simulink model "LinkageC"  (R2025b)
settings: Solver=VariableStepAuto  StartTime=0  StopTime=numPeriods*T  RelTol=1e-3  AbsTol=1e-3
values from neighbouring files (symbols this model uses):
  A_G = 56.801    [LinkageGeometrySetUp.m]    (also in LinkageGeometrySetUp_imp.m = 55; LinkageGeometry_Fabio_ver.m = 20)
  alpha_0 = deg2rad(0.5)    [Iteration.m]    (also in Iteration_geometry.m; StartUp.m)
  alpha_stall_static = deg2rad(13)    [Iteration.m]    (also in Iteration_geometry.m; StartUp.m)
  AR = b^2/A    [LinkageGeometry_Modify.m]    (also in StartUp.m)
  Cd_cf = 1.5    [Iteration.m]    (also in Iteration_geometry.m; StartUp.m)
  CordOut = linspace(CordOut_root, CordOut_tip, WingSecNum_Out)    [LinkageGeometry_Modify.m]    (also in StartUp.m)
  D = 0;" newline      "    return;" newline      "end" newline      "q = 0.5*rho*Vmag^2;" newline      "D = q*S*CD;" newline      "L = q*S*CL;" newline      "    [build_wing_template.m]
  del_t = t_tot/(numSample)    [InputSetUp.m]
  eta_s = 0.90    (= 0.9)    [Iteration.m]    (also in Iteration_geometry.m; StartUp.m)
  InboardCord = 0.35*L_D/0.037    [LinkageGeometry_Modify.m]    (also in StartUp.m = 0.4)
  k_inboard = k * InboardCord/meanCord    [LinkageGeometry_Modify.m]    (also in StartUp.m = 12.5663706144)
  k_outboard = k * CordOut/meanCord    [LinkageGeometry_Modify.m]    (also in StartUp.m)
  Ka = 10    [StartUp3_control.m]
  Km = 73    [StartUp3_control.m]
  L_C = (3.589/1.5)*L_D    [LinkageGeometrySetUp.m]    (also in LinkageGeometrySetUp_imp.m = (9.37/3.7)*L_D; LinkageGeometry_Fabio_ver.m = 0.07885)
  L_C1 = (2.445/1.5)*L_D    [LinkageGeometrySetUp.m]    (also in LinkageGeometrySetUp_imp.m = (5.91/3.7)*L_D; LinkageGeometry_Fabio_ver.m = 0.04893)
  L_D = L_D_val(iter)    [Iteration_geometry.m]    (also in LinkageGeometry_Fabio_ver.m = 0.03019; StartUp.m = 0.037)
  L_EF = (1.494/1.5)*L_D    [LinkageGeometrySetUp.m]    (also in LinkageGeometrySetUp_imp.m = (4.468/3.7)*L_D; LinkageGeometry_Fabio_ver.m = 0.036)
  L_EG = (1.265/1.5)*L_D    [LinkageGeometrySetUp.m]    (also in LinkageGeometrySetUp_imp.m = L_C2; LinkageGeometry_Fabio_ver.m = 0.03)
  L_F = (16.189/1.5)*L_D    [LinkageGeometrySetUp.m]    (also in LinkageGeometrySetUp_imp.m = (39.93/3.7)*L_D; LinkageGeometry_Fabio_ver.m = 0.364)
  L_FH = (1.002/1.5)*L_D    [LinkageGeometrySetUp.m]    (also in LinkageGeometrySetUp_imp.m = (2.842/3.7)*L_D; LinkageGeometry_Fabio_ver.m = 0.02)
  L_Fl = (16.118/1.5)*L_D    [LinkageGeometrySetUp.m]    (also in LinkageGeometrySetUp_imp.m = L_F; LinkageGeometry_Fabio_ver.m = 0.364)
  L_Fp = (4.051/1.5)*L_D    [LinkageGeometrySetUp.m]    (also in LinkageGeometrySetUp_imp.m = (9.99/3.7)*L_D; LinkageGeometry_Fabio_ver.m = 0.14288)
  L_GH = (1.129/1.5)*L_D    [LinkageGeometrySetUp.m]    (also in LinkageGeometrySetUp_imp.m = (3.046/3.7)*L_D; LinkageGeometry_Fabio_ver.m = 0.016)
  L_t = 0.5/100    (= 0.005)    [LinkageGeometrySetUp.m]    (also in LinkageGeometrySetUp_imp.m; LinkageGeometry_Fabio_ver.m; LinkageGeometry_Modify.m)
  L_tip = (19.334/1.5)*L_D    [LinkageGeometrySetUp.m]    (also in LinkageGeometrySetUp_imp.m = (43/3.7)*L_D; LinkageGeometry_Fabio_ver.m = 0.55)
  M_in_i = M_in/WingSecNum_In    (= 0.0341666666667)    [StartUp.m]
  M_ser = 0.02    [StartUp.m]
  mu = 1.81e-5    (= 1.81e-05)    [Iteration.m]    (also in Iteration_geometry.m; StartUp.m)
  noise_freq_cutoff = 20*ang_freq    [InputSetUp.m]
  P_ref = 10    [StartUp3_control.m]
  phase_data_lookup = phase_data_lookup(1:(end-1))    [StartUp.m]
  pitch_data_lookup = pitch_ts.Data(1:numSampPerT)    [InputSetUp.m]
  pitch_gain = linspace(0.1, 1, WingSecNum_Out)    [InputSetUp.m]
  pitch_lookup_input = 1    [Iteration.m]    (also in Iteration_geometry.m; StartUp.m)
  pitch_mean = deg2rad(20)    [Iteration.m]    (also in Iteration_geometry.m; Iteration_speed.m; StartUp.m = deg2rad(1); StartUp3_control.m = deg2rad(1))
  rho = 1.225    [StartUp.m]
  SectionWidth_In = L_Inboard/WingSecNum_In    [LinkageGeometry_Modify.m]    (also in StartUp.m = (L_Inboard/WingSecNum_In)*0.6)
  SectionWidth_Out = L_outboard/WingSecNum_Out    [LinkageGeometry_Modify.m]    (also in StartUp.m)
  SpeedControlYes = 1    [StartUp3_control.m]
  TorqueLimit = 7.2    [StartUp3_control.m]
  U = 0.1    [Iteration.m]    (also in Iteration_geometry.m; StartUp.m)
  xi = 0.0    (= 0)    [Iteration.m]    (also in Iteration_geometry.m; StartUp.m)
undefined symbols (not defined in the file or in its folder): angle_data_lookup, DiscIntNeverNeededParam, magnitude, Pivot, X, Y, Z
libraries: sm_lib x1370, nesl_utility x916, simulink x478, cstblocks x78, simulink_extras x10, slpidlib x2
(part 53 of 57)

== matlab function LinkageC/Subsystem2/Parallelogram/WingSeg_In_2/1993dL&dT/AeroCalc ==
  data: dL output size=[1 1]; R input size=[3 3]; dT output size=[1 1]; h_dot input size=[1 1]; h_ddot input size=[1 1]; i input size=[1 1]; in input size=[1 1]; pitch_i input size=[1 1]; pitch_i_d input size=[1 1]; pitch_i_dd input size=[1 1]; pitch_mean parameter size=[1 1]; pitch_gain parameter; k_inboard parameter; k_outboard parameter; U parameter size=[1 1]; rho parameter size=[1 1]; AR parameter size=[1 1]; mu parameter size=[1 1]; xi parameter size=[1 1]; alpha_0 parameter size=[1 1]; alpha_stall_static parameter size=[1 1]; eta_s parameter size=[1 1]; Cd_cf parameter size=[1 1]; InboardCord parameter; CordOut parameter; SectionWidth_In parameter; SectionWidth_Out parameter size=[1 1]; stall_yes output
function [dL, dT, stall_yes] = fcn(R, h_dot, h_ddot, i, in , ...
    pitch_i,pitch_i_d,pitch_i_dd, pitch_mean, pitch_gain, ...
    k_inboard, k_outboard, ...
    U,rho, AR, mu, xi, alpha_0, alpha_stall_static, eta_s, Cd_cf, ...
    InboardCord,CordOut, SectionWidth_In,SectionWidth_Out) 
    % Notes:
    %   - wing root i = 1, wing tip i = wing section number
    %   - the smaller the i, the closer to the root
    % Parameters:
    %   - R = rotational matrix
    %   - h_dot = leading edge velocity (m/s)
    %   - pitch (may be inaccurate, but currently taken as w.r.t spar....)

    R = 1*R;  % rotation matrix (not yet used)
     
    % Simple steady state version (?):
    % V = [Vx, Vy, Vz];
    % Vmag = norm(V);
    % if Vmag < 1e-9
    %     Fx = 0; Fy = 0; Fz = 0; L = 0; D = 0;
    %     return;
    % end
    % q = 0.5*rho*Vmag^2;
    % D = q*S*CD;
    % L = q*S*CL;
    % % drag opposite velocity, lift along +y 
    % % U is in + z direction
    % u = (V+[0,0,U]) / Vmag; % normal vector for V direction relative to air
    % Fdrag = -D*u;
    % Flift = [0,L,0];
    % F = Fdrag + Flift;
    % Fx = F(1); Fy = F(2); Fz = F(3);


    % 1993 code start's here --------------------------------------------
    i = round(i);
    C_1 = 0.5*AR/(2.32+AR);
    C_2 = 0.181+0.772/AR;
    F_k = @(k)   1 - C_1 *(k.^2)./(k.^2 +C_2^2);
    G_k = @(k)   -C_1*C_2*k./(k.^2 +C_2^2);
    C_k = @(k)   F_k(k) + 1i*G_k(k);

    if (round(in) == 1)
        % when it's inboard wing
        dy = SectionWidth_In;
        cord_i = InboardCord;
        pitch_gain_i = 0;
        k_i = k_inboard;
        %C_k_Jones_i = C_k_Jones(k_inboard);
    else % in == 0
        % when it's outboard wing
        dy = SectionWidth_Out;
        cord_i = CordOut(i);
        pitch_gain_i = pitch_gain(i);
        k_i = k_outboard(i);
        %C_k_Jones_i = C_k_Jones(k_outboard(i));
    end

    % scaling the pitch angle
    pitch_mean_i = pitch_mean; % pitch mean is same for all. though not 
                               % shown in simulation for inboard arm
    pitch_i    = pitch_i   *pitch_gain_i;
    pitch_i_d  = pitch_i_d *pitch_gain_i;
    pitch_i_dd = pitch_i_dd*pitch_gain_i;

    w0_U = 2*(alpha_0 + pitch_mean_i)/ (2+AR);

    %all pitch values are in rad
    alpha_i = (h_dot * cos(pitch_i) ...
               + 0.75 * cord_i * pitch_i_d ...
               + U * (pitch_i - pitch_mean_i))/U;
        
    % Time derivative of alpha_i
    alpha_i_d = (h_ddot * cos(pitch_i) ...
            - h_dot * sin(pitch_i) * pitch_i_d ...
            + 0.75 * cord_i * pitch_i_dd ...
            + U * pitch_i_d ) / U;

    %alpha_prime = C_k_Jones_i*alpha_i - w0_U;
    % assume sinusoidal pitching, then:
    alpha_prime = (AR/(2+AR))*(F_k(k_i)*alpha_i + cord_i*G_k(k_i)*alpha_i_d/(2*U*k_i))- w0_U;
    %alpha_prime = alpha_i - w0_U;

    V_34_term1 = U*cos(pitch_i) - h_dot*sin(pitch_i);
    V_34_term2 = U*(alpha_prime+pitch_mean_i) - 0.5*cord_i*pitch_i_d;
    V_34 = sqrt(V_34_term1^2 + V_34_term2^2);

    Cn_y = 2 * pi * (alpha_prime + alpha_0 + pitch_mean_i);
   
    dNc = 0.5*rho*U*V_34*Cn_y*cord_i*dy;

    V_24_d =  U * alpha_i_d - 0.25 * cord_i * pitch_i_dd;
    dNa = 0.25*rho*pi*(cord_i^2)*V_24_d*dy;

    dN = dNa + dNc;

    % Eq. (17): chordwise force due to camber
    dD_camber = -2*pi*alpha_0*(alpha_prime + pitch_mean_i) ...
                * (rho*U*V_34/2) * cord_i * dy;

    % Eq. (18): leading-edge suction term
    dT_s = eta_s * 2*pi * ( alpha_prime + pitch_mean_i ...
          - (cord_i*pitch_i_d)/(4*U) )^2 ...
          * (rho*U*V_34/2) * cord_i * dy;
    
    % Eq. (19): viscous skin-friction drag
    % Eq. (20): tangential flow speed approximation
    V_x = U*cos(pitch_i) - h_dot*sin(pitch_i);
    
    Re_i   = rho * V_34 * cord_i / mu;
    c_df_i = 0.89 / (log10(Re_i)^2.58);
    dD_f = c_df_i * (rho*V_x^2/2) * cord_i * dy;
    
    % Eq. (21): total chordwise force
    dFx = dT_s - dD_camber - dD_f;
    
    % Eq. (22): dynamic stall angle
    alpha_stall = alpha_stall_static + xi * sqrt(abs(cord_i * pitch_i_d / (2*U)));

    % Eq. (23)
    stall_metric = alpha_prime + pitch_mean_i - 0.75 * (cord_i * pitch_i_d / U);
    stall_yes = stall_metric - alpha_stall; 
    if stall_yes > 0
        V_n = h_dot*cos(pitch_i) + 0.5*cord_i*pitch_i_d + U*sin(pitch_i);
        V_hat = sqrt(V_x^2 + V_n^2);
  
        dNc_sep = Cd_cf * 0.5 * rho * V_hat * V_n * cord_i * dy;
        dNa_sep = 0.5*dNa;

        dN = dNc_sep + dNa_sep;
        dFx = 0;  
    end
    
    dL = dN * cos(pitch_i) + dFx * sin(pitch_i);
    dT = dFx * cos(pitch_i) - dN * sin(pitch_i);
end

== matlab function LinkageC/Subsystem2/Parallelogram/WingSeg_In_3/1993dL&dT/AeroCalc ==
  data: dL output size=[1 1]; R input size=[3 3]; dT output size=[1 1]; h_dot input size=[1 1]; h_ddot input size=[1 1]; i input size=[1 1]; in input size=[1 1]; pitch_i input size=[1 1]; pitch_i_d input size=[1 1]; pitch_i_dd input size=[1 1]; pitch_mean parameter size=[1 1]; pitch_gain parameter; k_inboard parameter; k_outboard parameter; U parameter size=[1 1]; rho parameter size=[1 1]; AR parameter size=[1 1]; mu parameter size=[1 1]; xi parameter size=[1 1]; alpha_0 parameter size=[1 1]; alpha_stall_static parameter size=[1 1]; eta_s parameter size=[1 1]; Cd_cf parameter size=[1 1]; InboardCord parameter; CordOut parameter; SectionWidth_In parameter; SectionWidth_Out parameter size=[1 1]; stall_yes output
function [dL, dT, stall_yes] = fcn(R, h_dot, h_ddot, i, in , ...
    pitch_i,pitch_i_d,pitch_i_dd, pitch_mean, pitch_gain, ...
    k_inboard, k_outboard, ...
    U,rho, AR, mu, xi, alpha_0, alpha_stall_static, eta_s, Cd_cf, ...
    InboardCord,CordOut, SectionWidth_In,SectionWidth_Out) 
    % Notes:
    %   - wing root i = 1, wing tip i = wing section number
    %   - the smaller the i, the closer to the root
    % Parameters:
    %   - R = rotational matrix
    %   - h_dot = leading edge velocity (m/s)
    %   - pitch (may be inaccurate, but currently taken as w.r.t spar....)

    R = 1*R;  % rotation matrix (not yet used)
     
    % Simple steady state version (?):
    % V = [Vx, Vy, Vz];
    % Vmag = norm(V);
    % if Vmag < 1e-9
    %     Fx = 0; Fy = 0; Fz = 0; L = 0; D = 0;
    %     return;
    % end
    % q = 0.5*rho*Vmag^2;
    % D = q*S*CD;
    % L = q*S*CL;
    % % drag opposite velocity, lift along +y 
    % % U is in + z direction
    % u = (V+[0,0,U]) / Vmag; % normal vector for V direction relative to air
    % Fdrag = -D*u;
    % Flift = [0,L,0];
    % F = Fdrag + Flift;
    % Fx = F(1); Fy = F(2); Fz = F(3);


    % 1993 code start's here --------------------------------------------
    i = round(i);
    C_1 = 0.5*AR/(2.32+AR);
    C_2 = 0.181+0.772/AR;
    F_k = @(k)   1 - C_1 *(k.^2)./(k.^2 +C_2^2);
    G_k = @(k)   -C_1*C_2*k./(k.^2 +C_2^2);
    C_k = @(k)   F_k(k) + 1i*G_k(k);

    if (round(in) == 1)
        % when it's inboard wing
        dy = SectionWidth_In;
        cord_i = InboardCord;
        pitch_gain_i = 0;
        k_i = k_inboard;
        %C_k_Jones_i = C_k_Jones(k_inboard);
    else % in == 0
        % when it's outboard wing
        dy = SectionWidth_Out;
        cord_i = CordOut(i);
        pitch_gain_i = pitch_gain(i);
        k_i = k_outboard(i);
        %C_k_Jones_i = C_k_Jones(k_outboard(i));
    end

    % scaling the pitch angle
    pitch_mean_i = pitch_mean; % pitch mean is same for all. though not 
                               % shown in simulation for inboard arm
    pitch_i    = pitch_i   *pitch_gain_i;
    pitch_i_d  = pitch_i_d *pitch_gain_i;
    pitch_i_dd = pitch_i_dd*pitch_gain_i;

    w0_U = 2*(alpha_0 + pitch_mean_i)/ (2+AR);

    %all pitch values are in rad
    alpha_i = (h_dot * cos(pitch_i) ...
               + 0.75 * cord_i * pitch_i_d ...
               + U * (pitch_i - pitch_mean_i))/U;
        
    % Time derivative of alpha_i
    alpha_i_d = (h_ddot * cos(pitch_i) ...
            - h_dot * sin(pitch_i) * pitch_i_d ...
            + 0.75 * cord_i * pitch_i_dd ...
            + U * pitch_i_d ) / U;

    %alpha_prime = C_k_Jones_i*alpha_i - w0_U;
    % assume sinusoidal pitching, then:
    alpha_prime = (AR/(2+AR))*(F_k(k_i)*alpha_i + cord_i*G_k(k_i)*alpha_i_d/(2*U*k_i))- w0_U;
    %alpha_prime = alpha_i - w0_U;

    V_34_term1 = U*cos(pitch_i) - h_dot*sin(pitch_i);
    V_34_term2 = U*(alpha_prime+pitch_mean_i) - 0.5*cord_i*pitch_i_d;
    V_34 = sqrt(V_34_term1^2 + V_34_term2^2);

    Cn_y = 2 * pi * (alpha_prime + alpha_0 + pitch_mean_i);
   
    dNc = 0.5*rho*U*V_34*Cn_y*cord_i*dy;

    V_24_d =  U * alpha_i_d - 0.25 * cord_i * pitch_i_dd;
    dNa = 0.25*rho*pi*(cord_i^2)*V_24_d*dy;

    dN = dNa + dNc;

    % Eq. (17): chordwise force due to camber
    dD_camber = -2*pi*alpha_0*(alpha_prime + pitch_mean_i) ...
                * (rho*U*V_34/2) * cord_i * dy;

    % Eq. (18): leading-edge suction term
    dT_s = eta_s * 2*pi * ( alpha_prime + pitch_mean_i ...
          - (cord_i*pitch_i_d)/(4*U) )^2 ...
          * (rho*U*V_34/2) * cord_i * dy;
    
    % Eq. (19): viscous skin-friction drag
    % Eq. (20): tangential flow speed approximation
    V_x = U*cos(pitch_i) - h_dot*sin(pitch_i);
    
    Re_i   = rho * V_34 * cord_i / mu;
    c_df_i = 0.89 / (log10(Re_i)^2.58);
    dD_f = c_df_i * (rho*V_x^2/2) * cord_i * dy;
    
    % Eq. (21): total chordwise force
    dFx = dT_s - dD_camber - dD_f;
    
    % Eq. (22): dynamic stall angle
    alpha_stall = alpha_stall_static + xi * sqrt(abs(cord_i * pitch_i_d / (2*U)));

    % Eq. (23)
    stall_metric = alpha_prime + pitch_mean_i - 0.75 * (cord_i * pitch_i_d / U);
    stall_yes = stall_metric - alpha_stall; 
    if stall_yes > 0
        V_n = h_dot*cos(pitch_i) + 0.5*cord_i*pitch_i_d + U*sin(pitch_i);
        V_hat = sqrt(V_x^2 + V_n^2);
  
        dNc_sep = Cd_cf * 0.5 * rho * V_hat * V_n * cord_i * dy;
        dNa_sep = 0.5*dNa;

        dN = dNc_sep + dNa_sep;
        dFx = 0;  
    end
    
    dL = dN * cos(pitch_i) + dFx * sin(pitch_i);
    dT = dFx * cos(pitch_i) - dN * sin(pitch_i);
end

== matlab function LinkageC/Subsystem2/Parallelogram/WingSeg_In_4/1993dL&dT/AeroCalc ==
  data: dL output size=[1 1]; R input size=[3 3]; dT output size=[1 1]; h_dot input size=[1 1]; h_ddot input size=[1 1]; i input size=[1 1]; in input size=[1 1]; pitch_i input size=[1 1]; pitch_i_d input size=[1 1]; pitch_i_dd input size=[1 1]; pitch_mean parameter size=[1 1]; pitch_gain parameter; k_inboard parameter; k_outboard parameter; U parameter size=[1 1]; rho parameter size=[1 1]; AR parameter size=[1 1]; mu parameter size=[1 1]; xi parameter size=[1 1]; alpha_0 parameter size=[1 1]; alpha_stall_static parameter size=[1 1]; eta_s parameter size=[1 1]; Cd_cf parameter size=[1 1]; InboardCord parameter; CordOut parameter; SectionWidth_In parameter; SectionWidth_Out parameter size=[1 1]; stall_yes output
function [dL, dT, stall_yes] = fcn(R, h_dot, h_ddot, i, in , ...
    pitch_i,pitch_i_d,pitch_i_dd, pitch_mean, pitch_gain, ...
    k_inboard, k_outboard, ...
    U,rho, AR, mu, xi, alpha_0, alpha_stall_static, eta_s, Cd_cf, ...
    InboardCord,CordOut, SectionWidth_In,SectionWidth_Out) 
    % Notes:
    %   - wing root i = 1, wing tip i = wing section number
    %   - the smaller the i, the closer to the root
    % Parameters:
    %   - R = rotational matrix
    %   - h_dot = leading edge velocity (m/s)
    %   - pitch (may be inaccurate, but currently taken as w.r.t spar....)

    R = 1*R;  % rotation matrix (not yet used)
     
    % Simple steady state version (?):
    % V = [Vx, Vy, Vz];
    % Vmag = norm(V);
    % if Vmag < 1e-9
    %     Fx = 0; Fy = 0; Fz = 0; L = 0; D = 0;
    %     return;
    % end
    % q = 0.5*rho*Vmag^2;
    % D = q*S*CD;
    % L = q*S*CL;
    % % drag opposite velocity, lift along +y 
    % % U is in + z direction
    % u = (V+[0,0,U]) / Vmag; % normal vector for V direction relative to air
    % Fdrag = -D*u;
    % Flift = [0,L,0];
    % F = Fdrag + Flift;
    % Fx = F(1); Fy = F(2); Fz = F(3);


    % 1993 code start's here --------------------------------------------
    i = round(i);
    C_1 = 0.5*AR/(2.32+AR);
    C_2 = 0.181+0.772/AR;
    F_k = @(k)   1 - C_1 *(k.^2)./(k.^2 +C_2^2);
    G_k = @(k)   -C_1*C_2*k./(k.^2 +C_2^2);
    C_k = @(k)   F_k(k) + 1i*G_k(k);

    if (round(in) == 1)
        % when it's inboard wing
        dy = SectionWidth_In;
        cord_i = InboardCord;
        pitch_gain_i = 0;
        k_i = k_inboard;
        %C_k_Jones_i = C_k_Jones(k_inboard);
    else % in == 0
        % when it's outboard wing
        dy = SectionWidth_Out;
        cord_i = CordOut(i);
        pitch_gain_i = pitch_gain(i);
        k_i = k_outboard(i);
        %C_k_Jones_i = C_k_Jones(k_outboard(i));
    end

    % scaling the pitch angle
    pitch_mean_i = pitch_mean; % pitch mean is same for all. though not 
                               % shown in simulation for inboard arm
    pitch_i    = pitch_i   *pitch_gain_i;
    pitch_i_d  = pitch_i_d *pitch_gain_i;
    pitch_i_dd = pitch_i_dd*pitch_gain_i;

    w0_U = 2*(alpha_0 + pitch_mean_i)/ (2+AR);

    %all pitch values are in rad
    alpha_i = (h_dot * cos(pitch_i) ...
               + 0.75 * cord_i * pitch_i_d ...
               + U * (pitch_i - pitch_mean_i))/U;
        
    % Time derivative of alpha_i
    alpha_i_d = (h_ddot * cos(pitch_i) ...
            - h_dot * sin(pitch_i) * pitch_i_d ...
            + 0.75 * cord_i * pitch_i_dd ...
            + U * pitch_i_d ) / U;

    %alpha_prime = C_k_Jones_i*alpha_i - w0_U;
    % assume sinusoidal pitching, then:
    alpha_prime = (AR/(2+AR))*(F_k(k_i)*alpha_i + cord_i*G_k(k_i)*alpha_i_d/(2*U*k_i))- w0_U;
    %alpha_prime = alpha_i - w0_U;

    V_34_term1 = U*cos(pitch_i) - h_dot*sin(pitch_i);
    V_34_term2 = U*(alpha_prime+pitch_mean_i) - 0.5*cord_i*pitch_i_d;
    V_34 = sqrt(V_34_term1^2 + V_34_term2^2);

    Cn_y = 2 * pi * (alpha_prime + alpha_0 + pitch_mean_i);
   
    dNc = 0.5*rho*U*V_34*Cn_y*cord_i*dy;

    V_24_d =  U * alpha_i_d - 0.25 * cord_i * pitch_i_dd;
    dNa = 0.25*rho*pi*(cord_i^2)*V_24_d*dy;

    dN = dNa + dNc;

    % Eq. (17): chordwise force due to camber
    dD_camber = -2*pi*alpha_0*(alpha_prime + pitch_mean_i) ...
                * (rho*U*V_34/2) * cord_i * dy;

    % Eq. (18): leading-edge suction term
    dT_s = eta_s * 2*pi * ( alpha_prime + pitch_mean_i ...
          - (cord_i*pitch_i_d)/(4*U) )^2 ...
          * (rho*U*V_34/2) * cord_i * dy;
    
    % Eq. (19): viscous skin-friction drag
    % Eq. (20): tangential flow speed approximation
    V_x = U*cos(pitch_i) - h_dot*sin(pitch_i);
    
    Re_i   = rho * V_34 * cord_i / mu;
    c_df_i = 0.89 / (log10(Re_i)^2.58);
    dD_f = c_df_i * (rho*V_x^2/2) * cord_i * dy;
    
    % Eq. (21): total chordwise force
    dFx = dT_s - dD_camber - dD_f;
    
    % Eq. (22): dynamic stall angle
    alpha_stall = alpha_stall_static + xi * sqrt(abs(cord_i * pitch_i_d / (2*U)));

    % Eq. (23)
    stall_metric = alpha_prime + pitch_mean_i - 0.75 * (cord_i * pitch_i_d / U);
    stall_yes = stall_metric - alpha_stall; 
    if stall_yes > 0
        V_n = h_dot*cos(pitch_i) + 0.5*cord_i*pitch_i_d + U*sin(pitch_i);
        V_hat = sqrt(V_x^2 + V_n^2);
  
        dNc_sep = Cd_cf * 0.5 * rho * V_hat * V_n * cord_i * dy;
        dNa_sep = 0.5*dNa;

        dN = dNc_sep + dNa_sep;
        dFx = 0;  
    end
    
    dL = dN * cos(pitch_i) + dFx * sin(pitch_i);
    dT = dFx * cos(pitch_i) - dN * sin(pitch_i);
end

== matlab function LinkageC/Subsystem2/Parallelogram/WingSeg_In_5/1993dL&dT/AeroCalc ==
  data: dL output size=[1 1]; R input size=[3 3]; dT output size=[1 1]; h_dot input size=[1 1]; h_ddot input size=[1 1]; i input size=[1 1]; in input size=[1 1]; pitch_i input size=[1 1]; pitch_i_d input size=[1 1]; pitch_i_dd input size=[1 1]; pitch_mean parameter size=[1 1]; pitch_gain parameter; k_inboard parameter; k_outboard parameter; U parameter size=[1 1]; rho parameter size=[1 1]; AR parameter size=[1 1]; mu parameter size=[1 1]; xi parameter size=[1 1]; alpha_0 parameter size=[1 1]; alpha_stall_static parameter size=[1 1]; eta_s parameter size=[1 1]; Cd_cf parameter size=[1 1]; InboardCord parameter; CordOut parameter; SectionWidth_In parameter; SectionWidth_Out parameter size=[1 1]; stall_yes output
function [dL, dT, stall_yes] = fcn(R, h_dot, h_ddot, i, in , ...
    pitch_i,pitch_i_d,pitch_i_dd, pitch_mean, pitch_gain, ...
    k_inboard, k_outboard, ...
    U,rho, AR, mu, xi, alpha_0, alpha_stall_static, eta_s, Cd_cf, ...
    InboardCord,CordOut, SectionWidth_In,SectionWidth_Out) 
    % Notes:
    %   - wing root i = 1, wing tip i = wing section number
    %   - the smaller the i, the closer to the root
    % Parameters:
    %   - R = rotational matrix
    %   - h_dot = leading edge velocity (m/s)
    %   - pitch (may be inaccurate, but currently taken as w.r.t spar....)

    R = 1*R;  % rotation matrix (not yet used)
     
    % Simple steady state version (?):
    % V = [Vx, Vy, Vz];
    % Vmag = norm(V);
    % if Vmag < 1e-9
    %     Fx = 0; Fy = 0; Fz = 0; L = 0; D = 0;
    %     return;
    % end
    % q = 0.5*rho*Vmag^2;
    % D = q*S*CD;
    % L = q*S*CL;
    % % drag opposite velocity, lift along +y 
    % % U is in + z direction
    % u = (V+[0,0,U]) / Vmag; % normal vector for V direction relative to air
    % Fdrag = -D*u;
    % Flift = [0,L,0];
    % F = Fdrag + Flift;
    % Fx = F(1); Fy = F(2); Fz = F(3);


    % 1993 code start's here --------------------------------------------
    i = round(i);
    C_1 = 0.5*AR/(2.32+AR);
    C_2 = 0.181+0.772/AR;
    F_k = @(k)   1 - C_1 *(k.^2)./(k.^2 +C_2^2);
    G_k = @(k)   -C_1*C_2*k./(k.^2 +C_2^2);
    C_k = @(k)   F_k(k) + 1i*G_k(k);

    if (round(in) == 1)
        % when it's inboard wing
        dy = SectionWidth_In;
        cord_i = InboardCord;
        pitch_gain_i = 0;
        k_i = k_inboard;
        %C_k_Jones_i = C_k_Jones(k_inboard);
    else % in == 0
        % when it's outboard wing
        dy = SectionWidth_Out;
        cord_i = CordOut(i);
        pitch_gain_i = pitch_gain(i);
        k_i = k_outboard(i);
        %C_k_Jones_i = C_k_Jones(k_outboard(i));
    end

    % scaling the pitch angle
    pitch_mean_i = pitch_mean; % pitch mean is same for all. though not 
                               % shown in simulation for inboard arm
    pitch_i    = pitch_i   *pitch_gain_i;
    pitch_i_d  = pitch_i_d *pitch_gain_i;
    pitch_i_dd = pitch_i_dd*pitch_gain_i;

    w0_U = 2*(alpha_0 + pitch_mean_i)/ (2+AR);

    %all pitch values are in rad
    alpha_i = (h_dot * cos(pitch_i) ...
               + 0.75 * cord_i * pitch_i_d ...
               + U * (pitch_i - pitch_mean_i))/U;
        
    % Time derivative of alpha_i
    alpha_i_d = (h_ddot * cos(pitch_i) ...
            - h_dot * sin(pitch_i) * pitch_i_d ...
            + 0.75 * cord_i * pitch_i_dd ...
            + U * pitch_i_d ) / U;

    %alpha_prime = C_k_Jones_i*alpha_i - w0_U;
    % assume sinusoidal pitching, then:
    alpha_prime = (AR/(2+AR))*(F_k(k_i)*alpha_i + cord_i*G_k(k_i)*alpha_i_d/(2*U*k_i))- w0_U;
    %alpha_prime = alpha_i - w0_U;

    V_34_term1 = U*cos(pitch_i) - h_dot*sin(pitch_i);
    V_34_term2 = U*(alpha_prime+pitch_mean_i) - 0.5*cord_i*pitch_i_d;
    V_34 = sqrt(V_34_term1^2 + V_34_term2^2);

    Cn_y = 2 * pi * (alpha_prime + alpha_0 + pitch_mean_i);
   
    dNc = 0.5*rho*U*V_34*Cn_y*cord_i*dy;

    V_24_d =  U * alpha_i_d - 0.25 * cord_i * pitch_i_dd;
    dNa = 0.25*rho*pi*(cord_i^2)*V_24_d*dy;

    dN = dNa + dNc;

    % Eq. (17): chordwise force due to camber
    dD_camber = -2*pi*alpha_0*(alpha_prime + pitch_mean_i) ...
                * (rho*U*V_34/2) * cord_i * dy;

    % Eq. (18): leading-edge suction term
    dT_s = eta_s * 2*pi * ( alpha_prime + pitch_mean_i ...
          - (cord_i*pitch_i_d)/(4*U) )^2 ...
          * (rho*U*V_34/2) * cord_i * dy;
    
    % Eq. (19): viscous skin-friction drag
    % Eq. (20): tangential flow speed approximation
    V_x = U*cos(pitch_i) - h_dot*sin(pitch_i);
    
    Re_i   = rho * V_34 * cord_i / mu;
    c_df_i = 0.89 / (log10(Re_i)^2.58);
    dD_f = c_df_i * (rho*V_x^2/2) * cord_i * dy;
    
    % Eq. (21): total chordwise force
    dFx = dT_s - dD_camber - dD_f;
    
    % Eq. (22): dynamic stall angle
    alpha_stall = alpha_stall_static + xi * sqrt(abs(cord_i * pitch_i_d / (2*U)));

    % Eq. (23)
    stall_metric = alpha_prime + pitch_mean_i - 0.75 * (cord_i * pitch_i_d / U);
    stall_yes = stall_metric - alpha_stall; 
    if stall_yes > 0
        V_n = h_dot*cos(pitch_i) + 0.5*cord_i*pitch_i_d + U*sin(pitch_i);
        V_hat = sqrt(V_x^2 + V_n^2);
  
        dNc_sep = Cd_cf * 0.5 * rho * V_hat * V_n * cord_i * dy;
        dNa_sep = 0.5*dNa;

        dN = dNc_sep + dNa_sep;
        dFx = 0;  
    end
    
    dL = dN * cos(pitch_i) + dFx * sin(pitch_i);
    dT = dFx * cos(pitch_i) - dN * sin(pitch_i);
end

== matlab function LinkageC/Subsystem2/Parallelogram/WingSeg_In_6/1993dL&dT/AeroCalc ==
  data: dL output size=[1 1]; R input size=[3 3]; dT output size=[1 1]; h_dot input size=[1 1]; h_ddot input size=[1 1]; i input size=[1 1]; in input size=[1 1]; pitch_i input size=[1 1]; pitch_i_d input size=[1 1]; pitch_i_dd input size=[1 1]; pitch_mean parameter size=[1 1]; pitch_gain parameter; k_inboard parameter; k_outboard parameter; U parameter size=[1 1]; rho parameter size=[1 1]; AR parameter size=[1 1]; mu parameter size=[1 1]; xi parameter size=[1 1]; alpha_0 parameter size=[1 1]; alpha_stall_static parameter size=[1 1]; eta_s parameter size=[1 1]; Cd_cf parameter size=[1 1]; InboardCord parameter; CordOut parameter; SectionWidth_In parameter; SectionWidth_Out parameter size=[1 1]; stall_yes output
function [dL, dT, stall_yes] = fcn(R, h_dot, h_ddot, i, in , ...
    pitch_i,pitch_i_d,pitch_i_dd, pitch_mean, pitch_gain, ...
    k_inboard, k_outboard, ...
    U,rho, AR, mu, xi, alpha_0, alpha_stall_static, eta_s, Cd_cf, ...
    InboardCord,CordOut, SectionWidth_In,SectionWidth_Out) 
    % Notes:
    %   - wing root i = 1, wing tip i = wing section number
    %   - the smaller the i, the closer to the root
    % Parameters:
    %   - R = rotational matrix
    %   - h_dot = leading edge velocity (m/s)
    %   - pitch (may be inaccurate, but currently taken as w.r.t spar....)

    R = 1*R;  % rotation matrix (not yet used)
     
    % Simple steady state version (?):
    % V = [Vx, Vy, Vz];
    % Vmag = norm(V);
    % if Vmag < 1e-9
    %     Fx = 0; Fy = 0; Fz = 0; L = 0; D = 0;
    %     return;
    % end
    % q = 0.5*rho*Vmag^2;
    % D = q*S*CD;
    % L = q*S*CL;
    % % drag opposite velocity, lift along +y 
    % % U is in + z direction
    % u = (V+[0,0,U]) / Vmag; % normal vector for V direction relative to air
    % Fdrag = -D*u;
    % Flift = [0,L,0];
    % F = Fdrag + Flift;
    % Fx = F(1); Fy = F(2); Fz = F(3);


    % 1993 code start's here --------------------------------------------
    i = round(i);
    C_1 = 0.5*AR/(2.32+AR);
    C_2 = 0.181+0.772/AR;
    F_k = @(k)   1 - C_1 *(k.^2)./(k.^2 +C_2^2);
    G_k = @(k)   -C_1*C_2*k./(k.^2 +C_2^2);
    C_k = @(k)   F_k(k) + 1i*G_k(k);

    if (round(in) == 1)
        % when it's inboard wing
        dy = SectionWidth_In;
        cord_i = InboardCord;
        pitch_gain_i = 0;
        k_i = k_inboard;
        %C_k_Jones_i = C_k_Jones(k_inboard);
    else % in == 0
        % when it's outboard wing
        dy = SectionWidth_Out;
        cord_i = CordOut(i);
        pitch_gain_i = pitch_gain(i);
        k_i = k_outboard(i);
        %C_k_Jones_i = C_k_Jones(k_outboard(i));
    end

    % scaling the pitch angle
    pitch_mean_i = pitch_mean; % pitch mean is same for all. though not 
                               % shown in simulation for inboard arm
    pitch_i    = pitch_i   *pitch_gain_i;
    pitch_i_d  = pitch_i_d *pitch_gain_i;
    pitch_i_dd = pitch_i_dd*pitch_gain_i;

    w0_U = 2*(alpha_0 + pitch_mean_i)/ (2+AR);

    %all pitch values are in rad
    alpha_i = (h_dot * cos(pitch_i) ...
               + 0.75 * cord_i * pitch_i_d ...
               + U * (pitch_i - pitch_mean_i))/U;
        
    % Time derivative of alpha_i
    alpha_i_d = (h_ddot * cos(pitch_i) ...
            - h_dot * sin(pitch_i) * pitch_i_d ...
            + 0.75 * cord_i * pitch_i_dd ...
            + U * pitch_i_d ) / U;

    %alpha_prime = C_k_Jones_i*alpha_i - w0_U;
    % assume sinusoidal pitching, then:
    alpha_prime = (AR/(2+AR))*(F_k(k_i)*alpha_i + cord_i*G_k(k_i)*alpha_i_d/(2*U*k_i))- w0_U;
    %alpha_prime = alpha_i - w0_U;

    V_34_term1 = U*cos(pitch_i) - h_dot*sin(pitch_i);
    V_34_term2 = U*(alpha_prime+pitch_mean_i) - 0.5*cord_i*pitch_i_d;
    V_34 = sqrt(V_34_term1^2 + V_34_term2^2);

    Cn_y = 2 * pi * (alpha_prime + alpha_0 + pitch_mean_i);
   
    dNc = 0.5*rho*U*V_34*Cn_y*cord_i*dy;

    V_24_d =  U * alpha_i_d - 0.25 * cord_i * pitch_i_dd;
    dNa = 0.25*rho*pi*(cord_i^2)*V_24_d*dy;

    dN = dNa + dNc;

    % Eq. (17): chordwise force due to camber
    dD_camber = -2*pi*alpha_0*(alpha_prime + pitch_mean_i) ...
                * (rho*U*V_34/2) * cord_i * dy;

    % Eq. (18): leading-edge suction term
    dT_s = eta_s * 2*pi * ( alpha_prime + pitch_mean_i ...
          - (cord_i*pitch_i_d)/(4*U) )^2 ...
          * (rho*U*V_34/2) * cord_i * dy;
    
    % Eq. (19): viscous skin-friction drag
    % Eq. (20): tangential flow speed approximation
    V_x = U*cos(pitch_i) - h_dot*sin(pitch_i);
    
    Re_i   = rho * V_34 * cord_i / mu;
    c_df_i = 0.89 / (log10(Re_i)^2.58);
    dD_f = c_df_i * (rho*V_x^2/2) * cord_i * dy;
    
    % Eq. (21): total chordwise force
    dFx = dT_s - dD_camber - dD_f;
    
    % Eq. (22): dynamic stall angle
    alpha_stall = alpha_stall_static + xi * sqrt(abs(cord_i * pitch_i_d / (2*U)));

    % Eq. (23)
    stall_metric = alpha_prime + pitch_mean_i - 0.75 * (cord_i * pitch_i_d / U);
    stall_yes = stall_metric - alpha_stall; 
    if stall_yes > 0
        V_n = h_dot*cos(pitch_i) + 0.5*cord_i*pitch_i_d + U*sin(pitch_i);
        V_hat = sqrt(V_x^2 + V_n^2);
  
        dNc_sep = Cd_cf * 0.5 * rho * V_hat * V_n * cord_i * dy;
        dNa_sep = 0.5*dNa;

        dN = dNc_sep + dNa_sep;
        dFx = 0;  
    end
    
    dL = dN * cos(pitch_i) + dFx * sin(pitch_i);
    dT = dFx * cos(pitch_i) - dN * sin(pitch_i);
end

== matlab function LinkageC/Subsystem2/Wing Tip/WingSeg_Out_1/1993dL&dT/AeroCalc ==
  data: dL output size=[1 1]; R input size=[3 3]; dT output size=[1 1]; h_dot input size=[1 1]; h_ddot input size=[1 1]; i input size=[1 1]; in input size=[1 1]; pitch_i input size=[1 1]; pitch_i_d input size=[1 1]; pitch_i_dd input size=[1 1]; pitch_mean parameter size=[1 1]; pitch_gain parameter; k_inboard parameter; k_outboard parameter; U parameter size=[1 1]; rho parameter size=[1 1]; AR parameter size=[1 1]; mu parameter size=[1 1]; xi parameter size=[1 1]; alpha_0 parameter size=[1 1]; alpha_stall_static parameter size=[1 1]; eta_s parameter size=[1 1]; Cd_cf parameter size=[1 1]; InboardCord parameter; CordOut parameter; SectionWidth_In parameter; SectionWidth_Out parameter size=[1 1]; stall_yes output
function [dL, dT, stall_yes] = fcn(R, h_dot, h_ddot, i, in , ...
    pitch_i,pitch_i_d,pitch_i_dd, pitch_mean, pitch_gain, ...
    k_inboard, k_outboard, ...
    U,rho, AR, mu, xi, alpha_0, alpha_stall_static, eta_s, Cd_cf, ...
    InboardCord,CordOut, SectionWidth_In,SectionWidth_Out) 
    % Notes:
    %   - wing root i = 1, wing tip i = wing section number
    %   - the smaller the i, the closer to the root
    % Parameters:
    %   - R = rotational matrix
    %   - h_dot = leading edge velocity (m/s)
    %   - pitch (may be inaccurate, but currently taken as w.r.t spar....)

    R = 1*R;  % rotation matrix (not yet used)
     
    % Simple steady state version (?):
    % V = [Vx, Vy, Vz];
    % Vmag = norm(V);
    % if Vmag < 1e-9
    %     Fx = 0; Fy = 0; Fz = 0; L = 0; D = 0;
    %     return;
    % end
    % q = 0.5*rho*Vmag^2;
    % D = q*S*CD;
    % L = q*S*CL;
    % % drag opposite velocity, lift along +y 
    % % U is in + z direction
    % u = (V+[0,0,U]) / Vmag; % normal vector for V direction relative to air
    % Fdrag = -D*u;
    % Flift = [0,L,0];
    % F = Fdrag + Flift;
    % Fx = F(1); Fy = F(2); Fz = F(3);


    % 1993 code start's here --------------------------------------------
    i = round(i);
    C_1 = 0.5*AR/(2.32+AR);
    C_2 = 0.181+0.772/AR;
    F_k = @(k)   1 - C_1 *(k.^2)./(k.^2 +C_2^2);
    G_k = @(k)   -C_1*C_2*k./(k.^2 +C_2^2);
    C_k = @(k)   F_k(k) + 1i*G_k(k);

    if (round(in) == 1)
        % when it's inboard wing
        dy = SectionWidth_In;
        cord_i = InboardCord;
        pitch_gain_i = 0;
        k_i = k_inboard;
        %C_k_Jones_i = C_k_Jones(k_inboard);
    else % in == 0
        % when it's outboard wing
        dy = SectionWidth_Out;
        cord_i = CordOut(i);
        pitch_gain_i = pitch_gain(i);
        k_i = k_outboard(i);
        %C_k_Jones_i = C_k_Jones(k_outboard(i));
    end

    % scaling the pitch angle
    pitch_mean_i = pitch_mean; % pitch mean is same for all. though not 
                               % shown in simulation for inboard arm
    pitch_i    = pitch_i   *pitch_gain_i;
    pitch_i_d  = pitch_i_d *pitch_gain_i;
    pitch_i_dd = pitch_i_dd*pitch_gain_i;

    w0_U = 2*(alpha_0 + pitch_mean_i)/ (2+AR);

    %all pitch values are in rad
    alpha_i = (h_dot * cos(pitch_i) ...
               + 0.75 * cord_i * pitch_i_d ...
               + U * (pitch_i - pitch_mean_i))/U;
        
    % Time derivative of alpha_i
    alpha_i_d = (h_ddot * cos(pitch_i) ...
            - h_dot * sin(pitch_i) * pitch_i_d ...
            + 0.75 * cord_i * pitch_i_dd ...
            + U * pitch_i_d ) / U;

    %alpha_prime = C_k_Jones_i*alpha_i - w0_U;
    % assume sinusoidal pitching, then:
    alpha_prime = (AR/(2+AR))*(F_k(k_i)*alpha_i + cord_i*G_k(k_i)*alpha_i_d/(2*U*k_i))- w0_U;
    %alpha_prime = alpha_i - w0_U;

    V_34_term1 = U*cos(pitch_i) - h_dot*sin(pitch_i);
    V_34_term2 = U*(alpha_prime+pitch_mean_i) - 0.5*cord_i*pitch_i_d;
    V_34 = sqrt(V_34_term1^2 + V_34_term2^2);

    Cn_y = 2 * pi * (alpha_prime + alpha_0 + pitch_mean_i);
   
    dNc = 0.5*rho*U*V_34*Cn_y*cord_i*dy;

    V_24_d =  U * alpha_i_d - 0.25 * cord_i * pitch_i_dd;
    dNa = 0.25*rho*pi*(cord_i^2)*V_24_d*dy;

    dN = dNa + dNc;

    % Eq. (17): chordwise force due to camber
    dD_camber = -2*pi*alpha_0*(alpha_prime + pitch_mean_i) ...
                * (rho*U*V_34/2) * cord_i * dy;

    % Eq. (18): leading-edge suction term
    dT_s = eta_s * 2*pi * ( alpha_prime + pitch_mean_i ...
          - (cord_i*pitch_i_d)/(4*U) )^2 ...
          * (rho*U*V_34/2) * cord_i * dy;
    
    % Eq. (19): viscous skin-friction drag
    % Eq. (20): tangential flow speed approximation
    V_x = U*cos(pitch_i) - h_dot*sin(pitch_i);
    
    Re_i   = rho * V_34 * cord_i / mu;
    c_df_i = 0.89 / (log10(Re_i)^2.58);
    dD_f = c_df_i * (rho*V_x^2/2) * cord_i * dy;
    
    % Eq. (21): total chordwise force
    dFx = dT_s - dD_camber - dD_f;
    
    % Eq. (22): dynamic stall angle
    alpha_stall = alpha_stall_static + xi * sqrt(abs(cord_i * pitch_i_d / (2*U)));

    % Eq. (23)
    stall_metric = alpha_prime + pitch_mean_i - 0.75 * (cord_i * pitch_i_d / U);
    stall_yes = stall_metric - alpha_stall; 
    if stall_yes > 0
        V_n = h_dot*cos(pitch_i) + 0.5*cord_i*pitch_i_d + U*sin(pitch_i);
        V_hat = sqrt(V_x^2 + V_n^2);
  
        dNc_sep = Cd_cf * 0.5 * rho * V_hat * V_n * cord_i * dy;
        dNa_sep = 0.5*dNa;

        dN = dNc_sep + dNa_sep;
        dFx = 0;  
    end
    
    dL = dN * cos(pitch_i) + dFx * sin(pitch_i);
    dT = dFx * cos(pitch_i) - dN * sin(pitch_i);
end

== matlab function LinkageC/Subsystem2/Wing Tip/WingSeg_Out_2/1993dL&dT/AeroCalc ==
  data: dL output size=[1 1]; R input size=[3 3]; dT output size=[1 1]; h_dot input size=[1 1]; h_ddot input size=[1 1]; i input size=[1 1]; in input size=[1 1]; pitch_i input size=[1 1]; pitch_i_d input size=[1 1]; pitch_i_dd input size=[1 1]; pitch_mean parameter size=[1 1]; pitch_gain parameter; k_inboard parameter; k_outboard parameter; U parameter size=[1 1]; rho parameter size=[1 1]; AR parameter size=[1 1]; mu parameter size=[1 1]; xi parameter size=[1 1]; alpha_0 parameter size=[1 1]; alpha_stall_static parameter size=[1 1]; eta_s parameter size=[1 1]; Cd_cf parameter size=[1 1]; InboardCord parameter; CordOut parameter; SectionWidth_In parameter; SectionWidth_Out parameter size=[1 1]; stall_yes output
function [dL, dT, stall_yes] = fcn(R, h_dot, h_ddot, i, in , ...
    pitch_i,pitch_i_d,pitch_i_dd, pitch_mean, pitch_gain, ...
    k_inboard, k_outboard, ...
    U,rho, AR, mu, xi, alpha_0, alpha_stall_static, eta_s, Cd_cf, ...
    InboardCord,CordOut, SectionWidth_In,SectionWidth_Out) 
    % Notes:
    %   - wing root i = 1, wing tip i = wing section number
    %   - the smaller the i, the closer to the root
    % Parameters:
    %   - R = rotational matrix
    %   - h_dot = leading edge velocity (m/s)
    %   - pitch (may be inaccurate, but currently taken as w.r.t spar....)

    R = 1*R;  % rotation matrix (not yet used)
     
    % Simple steady state version (?):
    % V = [Vx, Vy, Vz];
    % Vmag = norm(V);
    % if Vmag < 1e-9
    %     Fx = 0; Fy = 0; Fz = 0; L = 0; D = 0;
    %     return;
    % end
    % q = 0.5*rho*Vmag^2;
    % D = q*S*CD;
    % L = q*S*CL;
    % % drag opposite velocity, lift along +y 
    % % U is in + z direction
    % u = (V+[0,0,U]) / Vmag; % normal vector for V direction relative to air
    % Fdrag = -D*u;
    % Flift = [0,L,0];
    % F = Fdrag + Flift;
    % Fx = F(1); Fy = F(2); Fz = F(3);


    % 1993 code start's here --------------------------------------------
    i = round(i);
    C_1 = 0.5*AR/(2.32+AR);
    C_2 = 0.181+0.772/AR;
    F_k = @(k)   1 - C_1 *(k.^2)./(k.^2 +C_2^2);
    G_k = @(k)   -C_1*C_2*k./(k.^2 +C_2^2);
    C_k = @(k)   F_k(k) + 1i*G_k(k);

    if (round(in) == 1)
        % when it's inboard wing
        dy = SectionWidth_In;
        cord_i = InboardCord;
        pitch_gain_i = 0;
        k_i = k_inboard;
        %C_k_Jones_i = C_k_Jones(k_inboard);
    else % in == 0
        % when it's outboard wing
        dy = SectionWidth_Out;
        cord_i = CordOut(i);
        pitch_gain_i = pitch_gain(i);
        k_i = k_outboard(i);
        %C_k_Jones_i = C_k_Jones(k_outboard(i));
    end

    % scaling the pitch angle
    pitch_mean_i = pitch_mean; % pitch mean is same for all. though not 
                               % shown in simulation for inboard arm
    pitch_i    = pitch_i   *pitch_gain_i;
    pitch_i_d  = pitch_i_d *pitch_gain_i;
    pitch_i_dd = pitch_i_dd*pitch_gain_i;

    w0_U = 2*(alpha_0 + pitch_mean_i)/ (2+AR);

    %all pitch values are in rad
    alpha_i = (h_dot * cos(pitch_i) ...
               + 0.75 * cord_i * pitch_i_d ...
               + U * (pitch_i - pitch_mean_i))/U;
        
    % Time derivative of alpha_i
    alpha_i_d = (h_ddot * cos(pitch_i) ...
            - h_dot * sin(pitch_i) * pitch_i_d ...
            + 0.75 * cord_i * pitch_i_dd ...
            + U * pitch_i_d ) / U;

    %alpha_prime = C_k_Jones_i*alpha_i - w0_U;
    % assume sinusoidal pitching, then:
    alpha_prime = (AR/(2+AR))*(F_k(k_i)*alpha_i + cord_i*G_k(k_i)*alpha_i_d/(2*U*k_i))- w0_U;
    %alpha_prime = alpha_i - w0_U;

    V_34_term1 = U*cos(pitch_i) - h_dot*sin(pitch_i);
    V_34_term2 = U*(alpha_prime+pitch_mean_i) - 0.5*cord_i*pitch_i_d;
    V_34 = sqrt(V_34_term1^2 + V_34_term2^2);

    Cn_y = 2 * pi * (alpha_prime + alpha_0 + pitch_mean_i);
   
    dNc = 0.5*rho*U*V_34*Cn_y*cord_i*dy;

    V_24_d =  U * alpha_i_d - 0.25 * cord_i * pitch_i_dd;
    dNa = 0.25*rho*pi*(cord_i^2)*V_24_d*dy;

    dN = dNa + dNc;

    % Eq. (17): chordwise force due to camber
    dD_camber = -2*pi*alpha_0*(alpha_prime + pitch_mean_i) ...
                * (rho*U*V_34/2) * cord_i * dy;

    % Eq. (18): leading-edge suction term
    dT_s = eta_s * 2*pi * ( alpha_prime + pitch_mean_i ...
          - (cord_i*pitch_i_d)/(4*U) )^2 ...
          * (rho*U*V_34/2) * cord_i * dy;
    
    % Eq. (19): viscous skin-friction drag
    % Eq. (20): tangential flow speed approximation
    V_x = U*cos(pitch_i) - h_dot*sin(pitch_i);
    
    Re_i   = rho * V_34 * cord_i / mu;
    c_df_i = 0.89 / (log10(Re_i)^2.58);
    dD_f = c_df_i * (rho*V_x^2/2) * cord_i * dy;
    
    % Eq. (21): total chordwise force
    dFx = dT_s - dD_camber - dD_f;
    
    % Eq. (22): dynamic stall angle
    alpha_stall = alpha_stall_static + xi * sqrt(abs(cord_i * pitch_i_d / (2*U)));

    % Eq. (23)
    stall_metric = alpha_prime + pitch_mean_i - 0.75 * (cord_i * pitch_i_d / U);
    stall_yes = stall_metric - alpha_stall; 
    if stall_yes > 0
        V_n = h_dot*cos(pitch_i) + 0.5*cord_i*pitch_i_d + U*sin(pitch_i);
        V_hat = sqrt(V_x^2 + V_n^2);
  
        dNc_sep = Cd_cf * 0.5 * rho * V_hat * V_n * cord_i * dy;
        dNa_sep = 0.5*dNa;

        dN = dNc_sep + dNa_sep;
        dFx = 0;  
    end
    
    dL = dN * cos(pitch_i) + dFx * sin(pitch_i);
    dT = dFx * cos(pitch_i) - dN * sin(pitch_i);
end

== matlab function LinkageC/Plant(oldWorking)/Wing Tip/WingSeg_Out_1/1993dL&dT/AeroCalc ==
  data: dL output size=[1 1]; R input size=[3 3]; dT output size=[1 1]; h_dot input size=[1 1]; h_ddot input size=[1 1]; i input size=[1 1]; in input size=[1 1]; pitch_i input size=[1 1]; pitch_i_d input size=[1 1]; pitch_i_dd input size=[1 1]; pitch_mean parameter size=[1 1]; pitch_gain parameter; k_inboard parameter; k_outboard parameter; U parameter size=[1 1]; rho parameter size=[1 1]; AR parameter size=[1 1]; mu parameter size=[1 1]; xi parameter size=[1 1]; alpha_0 parameter size=[1 1]; alpha_stall_static parameter size=[1 1]; eta_s parameter size=[1 1]; Cd_cf parameter size=[1 1]; InboardCord parameter; CordOut parameter; SectionWidth_In parameter; SectionWidth_Out parameter size=[1 1]; stall_yes output
function [dL, dT, stall_yes] = fcn(R, h_dot, h_ddot, i, in , ...
    pitch_i,pitch_i_d,pitch_i_dd, pitch_mean, pitch_gain, ...
    k_inboard, k_outboard, ...
    U,rho, AR, mu, xi, alpha_0, alpha_stall_static, eta_s, Cd_cf, ...
    InboardCord,CordOut, SectionWidth_In,SectionWidth_Out) 
    % Notes:
    %   - wing root i = 1, wing tip i = wing section number
    %   - the smaller the i, the closer to the root
    % Parameters:
    %   - R = rotational matrix
    %   - h_dot = leading edge velocity (m/s)
    %   - pitch (may be inaccurate, but currently taken as w.r.t spar....)

    R = 1*R;  % rotation matrix (not yet used)
     
    % Simple steady state version (?):
    % V = [Vx, Vy, Vz];
    % Vmag = norm(V);
    % if Vmag < 1e-9
    %     Fx = 0; Fy = 0; Fz = 0; L = 0; D = 0;
    %     return;
    % end
    % q = 0.5*rho*Vmag^2;
    % D = q*S*CD;
    % L = q*S*CL;
    % % drag opposite velocity, lift along +y 
    % % U is in + z direction
    % u = (V+[0,0,U]) / Vmag; % normal vector for V direction relative to air
    % Fdrag = -D*u;
    % Flift = [0,L,0];
    % F = Fdrag + Flift;
    % Fx = F(1); Fy = F(2); Fz = F(3);


    % 1993 code start's here --------------------------------------------
    i = round(i);
    C_1 = 0.5*AR/(2.32+AR);
    C_2 = 0.181+0.772/AR;
    F_k = @(k)   1 - C_1 *(k.^2)./(k.^2 +C_2^2);
    G_k = @(k)   -C_1*C_2*k./(k.^2 +C_2^2);
    C_k = @(k)   F_k(k) + 1i*G_k(k);

    if (round(in) == 1)
        % when it's inboard wing
        dy = SectionWidth_In;
        cord_i = InboardCord;
        pitch_gain_i = 0;
        k_i = k_inboard;
        %C_k_Jones_i = C_k_Jones(k_inboard);
    else % in == 0
        % when it's outboard wing
        dy = SectionWidth_Out;
        cord_i = CordOut(i);
        pitch_gain_i = pitch_gain(i);
        k_i = k_outboard(i);
        %C_k_Jones_i = C_k_Jones(k_outboard(i));
    end

    % scaling the pitch angle
    pitch_mean_i = pitch_mean; % pitch mean is same for all. though not 
                               % shown in simulation for inboard arm
    pitch_i    = pitch_i   *pitch_gain_i;
    pitch_i_d  = pitch_i_d *pitch_gain_i;
    pitch_i_dd = pitch_i_dd*pitch_gain_i;

    w0_U = 2*(alpha_0 + pitch_mean_i)/ (2+AR);

    %all pitch values are in rad
    alpha_i = (h_dot * cos(pitch_i) ...
               + 0.75 * cord_i * pitch_i_d ...
               + U * (pitch_i - pitch_mean_i))/U;
        
    % Time derivative of alpha_i
    alpha_i_d = (h_ddot * cos(pitch_i) ...
            - h_dot * sin(pitch_i) * pitch_i_d ...
            + 0.75 * cord_i * pitch_i_dd ...
            + U * pitch_i_d ) / U;

    %alpha_prime = C_k_Jones_i*alpha_i - w0_U;
    % assume sinusoidal pitching, then:
    alpha_prime = (AR/(2+AR))*(F_k(k_i)*alpha_i + cord_i*G_k(k_i)*alpha_i_d/(2*U*k_i))- w0_U;
    %alpha_prime = alpha_i - w0_U;

    V_34_term1 = U*cos(pitch_i) - h_dot*sin(pitch_i);
    V_34_term2 = U*(alpha_prime+pitch_mean_i) - 0.5*cord_i*pitch_i_d;
    V_34 = sqrt(V_34_term1^2 + V_34_term2^2);

    Cn_y = 2 * pi * (alpha_prime + alpha_0 + pitch_mean_i);
   
    dNc = 0.5*rho*U*V_34*Cn_y*cord_i*dy;

    V_24_d =  U * alpha_i_d - 0.25 * cord_i * pitch_i_dd;
    dNa = 0.25*rho*pi*(cord_i^2)*V_24_d*dy;

    dN = dNa + dNc;

    % Eq. (17): chordwise force due to camber
    dD_camber = -2*pi*alpha_0*(alpha_prime + pitch_mean_i) ...
                * (rho*U*V_34/2) * cord_i * dy;

    % Eq. (18): leading-edge suction term
    dT_s = eta_s * 2*pi * ( alpha_prime + pitch_mean_i ...
          - (cord_i*pitch_i_d)/(4*U) )^2 ...
          * (rho*U*V_34/2) * cord_i * dy;
    
    % Eq. (19): viscous skin-friction drag
    % Eq. (20): tangential flow speed approximation
    V_x = U*cos(pitch_i) - h_dot*sin(pitch_i);
    
    Re_i   = rho * V_34 * cord_i / mu;
    c_df_i = 0.89 / (log10(Re_i)^2.58);
    dD_f = c_df_i * (rho*V_x^2/2) * cord_i * dy;
    
    % Eq. (21): total chordwise force
    dFx = dT_s - dD_camber - dD_f;
    
    % Eq. (22): dynamic stall angle
    alpha_stall = alpha_stall_static + xi * sqrt(abs(cord_i * pitch_i_d / (2*U)));

    % Eq. (23)
    stall_metric = alpha_prime + pitch_mean_i - 0.75 * (cord_i * pitch_i_d / U);
    stall_yes = stall_metric - alpha_stall; 
    if stall_yes > 0
        V_n = h_dot*cos(pitch_i) + 0.5*cord_i*pitch_i_d + U*sin(pitch_i);
        V_hat = sqrt(V_x^2 + V_n^2);
  
        dNc_sep = Cd_cf * 0.5 * rho * V_hat * V_n * cord_i * dy;
        dNa_sep = 0.5*dNa;

        dN = dNc_sep + dNa_sep;
        dFx = 0;  
    end
    
    dL = dN * cos(pitch_i) + dFx * sin(pitch_i);
    dT = dFx * cos(pitch_i) - dN * sin(pitch_i);
end
